simulink model "INtegrated_Simplified_Batteries_2"  (R2025a)
settings: Solver=ode113  StartTime=0.0  StopTime=20000  FixedStep=0.01  MaxStep=0.1  RelTol=1e-3
libraries: simulink x16, slpidlib x2, spsFirstOrderFilterLib x1
(part 2 of 3)

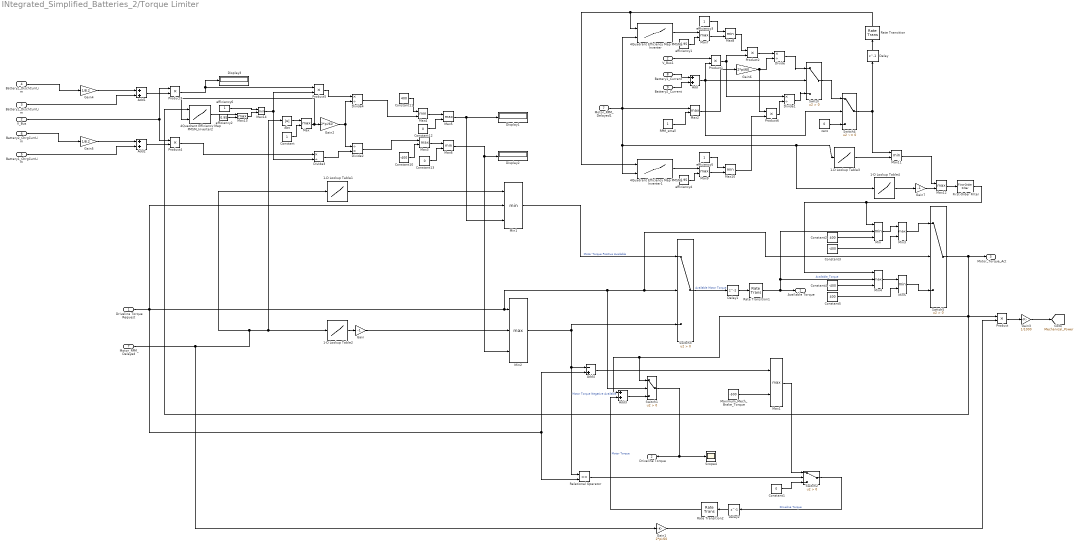
== system INtegrated_Simplified_Batteries_2/Torque Limiter ==
  Driveline Torque Request : Inport
  V_Bus : Inport  Port=2
  Battery1_DischCurrLim : Inport  Port=3
  Battery2_DischCurrLim : Inport  Port=4
  Battery1_ChrgCurrLim : Inport  Port=5
  Battery2_ChrgCurrLim : Inport  Port=6
  Motor_RPM_Delayed : Inport  Port=7
  Battery1_Current : Inport  Port=8
  Battery2_Current : Inport  Port=9
  1-D Lookup Table1 : Lookup_n-D  NumberOfTableDimensions=1  BreakpointsForDimension1=-19500:550:19500  Table=|  InternalRulePriority=Speed  RndMeth=Simplest
      | [5.617233286
      | 97.42737775
      | 101.4868518
      | 105.8188093
      | 110.4506091
      | 115.4133846
      | 120.7427184
      | 126.4794656
      | 132.6707681
      | 139.3713119
      | 146.6448989
      | 154.5664284
      | 163.2244193
      | 172.7242532
      | 183.1923898
      | 194.7819136
      | 207.6799304
      | 222.1175726
      | 238.3837585
      | 256.8444536
      | 277.9701878
      | 302.3762727
      | 330.8831267
      | 364.609506
      | 400
      | 400
      | 400
      | 400
      | 400
      | 400
      | 400
      | 400
      | 400
      | 400
      | 400
      | 400
      | 400
      | 400
      | 400
      | 400
      | 400
      | 400
      | 400
      | 400
      | 400
      | 400
      | 364.609506
      | 330.8831267
      | 302.3762727
      | 277.9701878
      | 256.8444536
      | 238.3837585
      | 222.1175726
      | 207.6799304
      | 194.7819136
      | 183.1923898
      | 172.7242532
      | 163.2244193
      | 154.5664284
      | 146.6448989
      | 139.3713119
      | 132.6707681
      | 126.4794656
      | 120.7427184
      | 115.4133846
      | 110.4506091
      | 105.8188093
      | 101.4868518
      | 97.42737775
      | 5.617233286
      | 0
      | ]
  1-D Lookup Table2 : Lookup_n-D  NumberOfTableDimensions=1  BreakpointsForDimension1=-19500:550:19500  Table=|  InternalRulePriority=Speed  RndMeth=Simplest
      | [5.617233286
      | 97.42737775
      | 101.4868518
      | 105.8188093
      | 110.4506091
      | 115.4133846
      | 120.7427184
      | 126.4794656
      | 132.6707681
      | 139.3713119
      | 146.6448989
      | 154.5664284
      | 163.2244193
      | 172.7242532
      | 183.1923898
      | 194.7819136
      | 207.6799304
      | 222.1175726
      | 238.3837585
      | 256.8444536
      | 277.9701878
      | 302.3762727
      | 330.8831267
      | 364.609506
      | 400
      | 400
      | 400
      | 400
      | 400
      | 400
      | 400
      | 400
      | 400
      | 400
      | 400
      | 400
      | 400
      | 400
      | 400
      | 400
      | 400
      | 400
      | 400
      | 400
      | 400
      | 400
      | 364.609506
      | 330.8831267
      | 302.3762727
      | 277.9701878
      | 256.8444536
      | 238.3837585
      | 222.1175726
      | 207.6799304
      | 194.7819136
      | 183.1923898
      | 172.7242532
      | 163.2244193
      | 154.5664284
      | 146.6448989
      | 139.3713119
      | 132.6707681
      | 126.4794656
      | 120.7427184
      | 115.4133846
      | 110.4506091
      | 105.8188093
      | 101.4868518
      | 97.42737775
      | 5.617233286
      | 0
      | ]
  1-D Lookup Table3 : Lookup_n-D  NumberOfTableDimensions=1  BreakpointsForDimension1=-19500:550:19500  Table=|  InternalRulePriority=Speed  RndMeth=Simplest
      | [5.617233286
      | 97.42737775
      | 101.4868518
      | 105.8188093
      | 110.4506091
      | 115.4133846
      | 120.7427184
      | 126.4794656
      | 132.6707681
      | 139.3713119
      | 146.6448989
      | 154.5664284
      | 163.2244193
      | 172.7242532
      | 183.1923898
      | 194.7819136
      | 207.6799304
      | 222.1175726
      | 238.3837585
      | 256.8444536
      | 277.9701878
      | 302.3762727
      | 330.8831267
      | 364.609506
      | 400
      | 400
      | 400
      | 400
      | 400
      | 400
      | 400
      | 400
      | 400
      | 400
      | 400
      | 400
      | 400
      | 400
      | 400
      | 400
      | 400
      | 400
      | 400
      | 400
      | 400
      | 400
      | 364.609506
      | 330.8831267
      | 302.3762727
      | 277.9701878
      | 256.8444536
      | 238.3837585
      | 222.1175726
      | 207.6799304
      | 194.7819136
      | 183.1923898
      | 172.7242532
      | 163.2244193
      | 154.5664284
      | 146.6448989
      | 139.3713119
      | 132.6707681
      | 126.4794656
      | 120.7427184
      | 115.4133846
      | 110.4506091
      | 105.8188093
      | 101.4868518
      | 97.42737775
      | 5.617233286
      | 0
      | ]
  1-D Lookup Table4 : Lookup_n-D  NumberOfTableDimensions=1  BreakpointsForDimension1=-19500:550:19500  Table=|  InternalRulePriority=Speed  RndMeth=Simplest
      | [5.617233286
      | 97.42737775
      | 101.4868518
      | 105.8188093
      | 110.4506091
      | 115.4133846
      | 120.7427184
      | 126.4794656
      | 132.6707681
      | 139.3713119
      | 146.6448989
      | 154.5664284
      | 163.2244193
      | 172.7242532
      | 183.1923898
      | 194.7819136
      | 207.6799304
      | 222.1175726
      | 238.3837585
      | 256.8444536
      | 277.9701878
      | 302.3762727
      | 330.8831267
      | 364.609506
      | 400
      | 400
      | 400
      | 400
      | 400
      | 400
      | 400
      | 400
      | 400
      | 400
      | 400
      | 400
      | 400
      | 400
      | 400
      | 400
      | 400
      | 400
      | 400
      | 400
      | 400
      | 400
      | 364.609506
      | 330.8831267
      | 302.3762727
      | 277.9701878
      | 256.8444536
      | 238.3837585
      | 222.1175726
      | 207.6799304
      | 194.7819136
      | 183.1923898
      | 172.7242532
      | 163.2244193
      | 154.5664284
      | 146.6448989
      | 139.3713119
      | 132.6707681
      | 126.4794656
      | 120.7427184
      | 115.4133846
      | 110.4506091
      | 105.8188093
      | 101.4868518
      | 97.42737775
      | 5.617233286
      | 0
      | ]
  4Quadrant Efficiency Map PMSM_Inverter : Lookup_n-D  BreakpointsForDimension1=-200:20:200  BreakpointsForDimension2=-16000:500:16000  Table=|  InterpMethod=Akima spline  InternalRulePriority=Speed  RndMeth=Simplest
      | [0.9785 0.9788 0.9792 0.9795 0.9799 0.9800 0.9800 0.9800 0.9800 0.9800 0.9800 0.9800 0.9800 0.9800 0.9800 0.9800 0.9800 0.9800 0.9800 0.9800 0.9800 0.9800 0.9800 0.9794 0.9781 0.9762 0.9737 0.9699 0.9641 0.9542 0.9347 0.8797 0.0000 0.8632 0.9301 0.9520 0.9628 0.9690 0.9730 0.9757 0.9776 0.9789 0.9799 0.9800 0.9800 0.9800 0.9800 0.9800 0.9800 0.9800 0.9800 0.9800 0.9800 0.9800 0.9800 0.9800 0.9800 0.9800 0.9800 0.9798 0.9794 0.9791 0.9787 0.9784 0.9780;
      | 0.9770 0.9774 0.9778 0.9782 0.9786 0.9790 0.9794 0.9797 0.9800 0.9800 0.9800 0.9800 0.9800 0.9800 0.9800 0.9800 0.9800 0.9800 0.9800 0.9800 0.9800 0.9800 0.9800 0.9800 0.9790 0.9774 0.9752 0.9719 0.9667 0.9578 0.9400 0.8894 0.0000 0.8756 0.9361 0.9559 0.9655 0.9711 0.9746 0.9769 0.9785 0.9797 0.9800 0.9800 0.9800 0.9800 0.9800 0.9800 0.9800 0.9800 0.9800 0.9800 0.9800 0.9800 0.9800 0.9797 0.9793 0.9789 0.9785 0.9781 0.9777 0.9773 0.9769 0.9764 0.9764;
      | 0.9750 0.9755 0.9760 0.9765 0.9769 0.9774 0.9779 0.9783 0.9787 0.9792 0.9796 0.9799 0.9800 0.9800 0.9800 0.9800 0.9800 0.9800 0.9800 0.9800 0.9800 0.9800 0.9800 0.9800 0.9797 0.9785 0.9766 0.9737 0.9691 0.9612 0.9452 0.8992 0.0000 0.8878 0.9420 0.9596 0.9681 0.9730 0.9760 0.9780 0.9793 0.9800 0.9800 0.9800 0.9800 0.9800 0.9800 0.9800 0.9800 0.9800 0.9800 0.9800 0.9799 0.9795 0.9791 0.9787 0.9783 0.9778 0.9774 0.9769 0.9764 0.9759 0.9754 0.9749 0.9743;
      | 0.9723 0.9729 0.9735 0.9741 0.9747 0.9752 0.9758 0.9764 0.9769 0.9774 0.9779 0.9784 0.9789 0.9793 0.9798 0.9800 0.9800 0.9800 0.9800 0.9800 0.9800 0.9800 0.9800 0.9800 0.9800 0.9793 0.9778 0.9754 0.9714 0.9645 0.9503 0.9089 0.0000 0.8998 0.9477 0.9632 0.9706 0.9747 0.9772 0.9788 0.9799 0.9800 0.9800 0.9800 0.9800 0.9800 0.9800 0.9800 0.9800 0.9798 0.9794 0.9789 0.9784 0.9779 0.9774 0.9769 0.9763 0.9758 0.9752 0.9746 0.9740 0.9734 0.9728 0.9722 0.9716;
      | 0.9687 0.9694 0.9701 0.9708 0.9715 0.9722 0.9729 0.9736 0.9743 0.9749 0.9756 0.9762 0.9768 0.9774 0.9780 0.9785 0.9790 0.9795 0.9799 0.9800 0.9800 0.9800 0.9800 0.9800 0.9800 0.9798 0.9786 0.9767 0.9735 0.9676 0.9553 0.9186 0.0000 0.9114 0.9532 0.9665 0.9728 0.9762 0.9782 0.9794 0.9800 0.9800 0.9800 0.9800 0.9800 0.9799 0.9795 0.9791 0.9786 0.9780 0.9775 0.9769 0.9763 0.9756 0.9750 0.9743 0.9736 0.9729 0.9722 0.9714 0.9707 0.9700 0.9692 0.9685 0.9677;
      | 0.9635 0.9644 0.9653 0.9661 0.9670 0.9679 0.9687 0.9696 0.9704 0.9712 0.9721 0.9729 0.9737 0.9744 0.9752 0.9759 0.9767 0.9773 0.9780 0.9786 0.9791 0.9795 0.9798 0.9800 0.9800 0.9798 0.9790 0.9777 0.9751 0.9703 0.9598 0.9280 0.0000 0.9224 0.9582 0.9694 0.9745 0.9772 0.9786 0.9793 0.9796 0.9796 0.9794 0.9791 0.9786 0.9781 0.9775 0.9768 0.9761 0.9753 0.9746 0.9738 0.9730 0.9721 0.9713 0.9704 0.9695 0.9686 0.9677 0.9668 0.9659 0.9649 0.9640 0.9631 0.9621;
      | 0.9557 0.9568 0.9579 0.9590 0.9601 0.9611 0.9622 0.9633 0.9644 0.9655 0.9666 0.9676 0.9687 0.9697 0.9707 0.9717 0.9727 0.9737 0.9746 0.9755 0.9763 0.9771 0.9777 0.9783 0.9787 0.9788 0.9786 0.9778 0.9761 0.9723 0.9638 0.9367 0.0000 0.9324 0.9624 0.9715 0.9755 0.9773 0.9781 0.9784 0.9782 0.9778 0.9772 0.9765 0.9757 0.9749 0.9739 0.9730 0.9720 0.9709 0.9699 0.9688 0.9677 0.9665 0.9654 0.9643 0.9631 0.9619 0.9608 0.9596 0.9584 0.9572 0.9560 0.9548 0.9536;
      | 0.9426 0.9440 0.9455 0.9470 0.9484 0.9499 0.9513 0.9528 0.9543 0.9557 0.9572 0.9586 0.9601 0.9615 0.9629 0.9643 0.9657 0.9671 0.9685 0.9698 0.9710 0.9723 0.9734 0.9745 0.9754 0.9761 0.9765 0.9764 0.9755 0.9730 0.9663 0.9438 0.0000 0.9404 0.9651 0.9722 0.9749 0.9759 0.9759 0.9755 0.9748 0.9738 0.9727 0.9715 0.9702 0.9688 0.9674 0.9660 0.9645 0.9630 0.9615 0.9600 0.9584 0.9568 0.9553 0.9537 0.9521 0.9505 0.9489 0.9472 0.9456 0.9440 0.9424 0.9407 0.9391;
      | 0.9171 0.9192 0.9213 0.9234 0.9256 0.9277 0.9298 0.9320 0.9341 0.9363 0.9384 0.9406 0.9427 0.9449 0.9470 0.9492 0.9513 0.9534 0.9555 0.9576 0.9597 0.9617 0.9637 0.9656 0.9673 0.9689 0.9703 0.9712 0.9714 0.9701 0.9653 0.9463 0.0000 0.9433 0.9640 0.9692 0.9706 0.9703 0.9694 0.9679 0.9662 0.9643 0.9623 0.9602 0.9580 0.9558 0.9535 0.9512 0.9488 0.9464 0.9441 0.9417 0.9392 0.9368 0.9344 0.9319 0.9295 0.9270 0.9245 0.9221 0.9196 0.9171 0.9146 0.9121 0.9096;
      | 0.8478 0.8514 0.8551 0.8588 0.8625 0.8662 0.8700 0.8738 0.8776 0.8815 0.8854 0.8893 0.8932 0.8972 0.9011 0.9051 0.9091 0.9132 0.9172 0.9213 0.9253 0.9293 0.9333 0.9372 0.9410 0.9447 0.9481 0.9510 0.9532 0.9537 0.9502 0.9309 0.0000 0.9257 0.9476 0.9515 0.9509 0.9485 0.9452 0.9415 0.9373 0.9330 0.9285 0.9239 0.9193 0.9145 0.9097 0.9049 0.9001 0.8952 0.8903 0.8854 0.8804 0.8755 0.8705 0.8655 0.8606 0.8556 0.8506 0.8456 0.8406 0.8356 0.8305 0.8255 0.8205;
      | 0.0000 0.0000 0.0000 0.0000 0.0000 0.0000 0.0000 0.0000 0.0000 0.0000 0.0000 0.0000 0.0000 0.0000 0.0000 0.0000 0.0000 0.0000 0.0000 0.0000 0.0000 0.0000 0.0000 0.0000 0.0000 0.0000 0.0000 0.0000 0.0000 0.0000 0.0000 0.0000 0.0000 0.0000 0.0000 0.0000 0.0000 0.0000 0.0000 0.0000 0.0000 0.0000 0.0000 0.0000 0.0000 0.0000 0.0000 0.0000 0.0000 0.0000 0.0000 0.0000 0.0000 0.0000 0.0000 0.0000 0.0000 0.0000 0.0000 0.0000 0.0000 0.0000 0.0000 0.0000 0.0000;
      | 0.8205 0.8255 0.8305 0.8356 0.8406 0.8456 0.8506 0.8556 0.8606 0.8655 0.8705 0.8755 0.8804 0.8854 0.8903 0.8952 0.9001 0.9049 0.9097 0.9145 0.9193 0.9239 0.9285 0.9330 0.9373 0.9415 0.9452 0.9485 0.9509 0.9515 0.9476 0.9257 0.0000 0.9309 0.9502 0.9537 0.9532 0.9510 0.9481 0.9447 0.9410 0.9372 0.9333 0.9293 0.9253 0.9213 0.9172 0.9132 0.9091 0.9051 0.9011 0.8972 0.8932 0.8893 0.8854 0.8815 0.8776 0.8738 0.8700 0.8662 0.8625 0.8588 0.8551 0.8514 0.8478;
      | 0.9096 0.9121 0.9146 0.9171 0.9196 0.9221 0.9245 0.9270 0.9295 0.9319 0.9344 0.9368 0.9392 0.9417 0.9441 0.9464 0.9488 0.9512 0.9535 0.9558 0.9580 0.9602 0.9623 0.9643 0.9662 0.9679 0.9694 0.9703 0.9706 0.9692 0.9640 0.9433 0.0000 0.9463 0.9653 0.9701 0.9714 0.9712 0.9703 0.9689 0.9673 0.9656 0.9637 0.9617 0.9597 0.9576 0.9555 0.9534 0.9513 0.9492 0.9470 0.9449 0.9427 0.9406 0.9384 0.9363 0.9341 0.9320 0.9298 0.9277 0.9256 0.9234 0.9213 0.9192 0.9171;
      | 0.9391 0.9407 0.9424 0.9440 0.9456 0.9472 0.9489 0.9505 0.9521 0.9537 0.9553 0.9568 0.9584 0.9600 0.9615 0.9630 0.9645 0.9660 0.9674 0.9688 0.9702 0.9715 0.9727 0.9738 0.9748 0.9755 0.9759 0.9759 0.9749 0.9722 0.9651 0.9404 0.0000 0.9438 0.9663 0.9730 0.9755 0.9764 0.9765 0.9761 0.9754 0.9745 0.9734 0.9723 0.9710 0.9698 0.9685 0.9671 0.9657 0.9643 0.9629 0.9615 0.9601 0.9586 0.9572 0.9557 0.9543 0.9528 0.9513 0.9499 0.9484 0.9470 0.9455 0.9440 0.9426;
      | 0.9536 0.9548 0.9560 0.9572 0.9584 0.9596 0.9608 0.9619 0.9631 0.9643 0.9654 0.9665 0.9677 0.9688 0.9699 0.9709 0.9720 0.9730 0.9739 0.9749 0.9757 0.9765 0.9772 0.9778 0.9782 0.9784 0.9781 0.9773 0.9755 0.9715 0.9624 0.9324 0.0000 0.9367 0.9638 0.9723 0.9761 0.9778 0.9786 0.9788 0.9787 0.9783 0.9777 0.9771 0.9763 0.9755 0.9746 0.9737 0.9727 0.9717 0.9707 0.9697 0.9687 0.9676 0.9666 0.9655 0.9644 0.9633 0.9622 0.9611 0.9601 0.9590 0.9579 0.9568 0.9557;
      | 0.9621 0.9631 0.9640 0.9649 0.9659 0.9668 0.9677 0.9686 0.9695 0.9704 0.9713 0.9721 0.9730 0.9738 0.9746 0.9753 0.9761 0.9768 0.9775 0.9781 0.9786 0.9791 0.9794 0.9796 0.9796 0.9793 0.9786 0.9772 0.9745 0.9694 0.9582 0.9224 0.0000 0.9280 0.9598 0.9703 0.9751 0.9777 0.9790 0.9798 0.9800 0.9800 0.9798 0.9795 0.9791 0.9786 0.9780 0.9773 0.9767 0.9759 0.9752 0.9744 0.9737 0.9729 0.9721 0.9712 0.9704 0.9696 0.9687 0.9679 0.9670 0.9661 0.9653 0.9644 0.9635;
      | 0.9677 0.9685 0.9692 0.9700 0.9707 0.9714 0.9722 0.9729 0.9736 0.9743 0.9750 0.9756 0.9763 0.9769 0.9775 0.9780 0.9786 0.9791 0.9795 0.9799 0.9800 0.9800 0.9800 0.9800 0.9800 0.9794 0.9782 0.9762 0.9728 0.9665 0.9532 0.9114 0.0000 0.9186 0.9553 0.9676 0.9735 0.9767 0.9786 0.9798 0.9800 0.9800 0.9800 0.9800 0.9800 0.9800 0.9799 0.9795 0.9790 0.9785 0.9780 0.9774 0.9768 0.9762 0.9756 0.9749 0.9743 0.9736 0.9729 0.9722 0.9715 0.9708 0.9701 0.9694 0.9687;
      | 0.9716 0.9722 0.9728 0.9734 0.9740 0.9746 0.9752 0.9758 0.9763 0.9769 0.9774 0.9779 0.9784 0.9789 0.9794 0.9798 0.9800 0.9800 0.9800 0.9800 0.9800 0.9800 0.9800 0.9800 0.9799 0.9788 0.9772 0.9747 0.9706 0.9632 0.9477 0.8998 0.0000 0.9089 0.9503 0.9645 0.9714 0.9754 0.9778 0.9793 0.9800 0.9800 0.9800 0.9800 0.9800 0.9800 0.9800 0.9800 0.9800 0.9800 0.9798 0.9793 0.9789 0.9784 0.9779 0.9774 0.9769 0.9764 0.9758 0.9752 0.9747 0.9741 0.9735 0.9729 0.9723;
      | 0.9743 0.9749 0.9754 0.9759 0.9764 0.9769 0.9774 0.9778 0.9783 0.9787 0.9791 0.9795 0.9799 0.9800 0.9800 0.9800 0.9800 0.9800 0.9800 0.9800 0.9800 0.9800 0.9800 0.9800 0.9793 0.9780 0.9760 0.9730 0.9681 0.9596 0.9420 0.8878 0.0000 0.8992 0.9452 0.9612 0.9691 0.9737 0.9766 0.9785 0.9797 0.9800 0.9800 0.9800 0.9800 0.9800 0.9800 0.9800 0.9800 0.9800 0.9800 0.9800 0.9800 0.9799 0.9796 0.9792 0.9787 0.9783 0.9779 0.9774 0.9769 0.9765 0.9760 0.9755 0.9750;
      | 0.9764 0.9769 0.9773 0.9777 0.9781 0.9785 0.9789 0.9793 0.9797 0.9800 0.9800 0.9800 0.9800 0.9800 0.9800 0.9800 0.9800 0.9800 0.9800 0.9800 0.9800 0.9800 0.9800 0.9797 0.9785 0.9769 0.9746 0.9711 0.9655 0.9559 0.9361 0.8756 0.0000 0.8894 0.9400 0.9578 0.9667 0.9719 0.9752 0.9774 0.9790 0.9800 0.9800 0.9800 0.9800 0.9800 0.9800 0.9800 0.9800 0.9800 0.9800 0.9800 0.9800 0.9800 0.9800 0.9800 0.9800 0.9797 0.9794 0.9790 0.9786 0.9782 0.9778 0.9774 0.9770;
      | 0.9780 0.9784 0.9787 0.9791 0.9794 0.9798 0.9800 0.9800 0.9800 0.9800 0.9800 0.9800 0.9800 0.9800 0.9800 0.9800 0.9800 0.9800 0.9800 0.9800 0.9800 0.9800 0.9799 0.9789 0.9776 0.9757 0.9730 0.9690 0.9628 0.9520 0.9301 0.8632 0.0000 0.8797 0.9347 0.9542 0.9641 0.9699 0.9737 0.9762 0.9781 0.9794 0.9800 0.9800 0.9800 0.9800 0.9800 0.9800 0.9800 0.9800 0.9800 0.9800 0.9800 0.9800 0.9800 0.9800 0.9800 0.9800 0.9800 0.9800 0.9799 0.9795 0.9792 0.9788 0.9785];
      settings: InputPortMap=u0,u1
  4Quadrant Efficiency Map PMSM_Inverter1 : Lookup_n-D  BreakpointsForDimension1=-200:20:200  BreakpointsForDimension2=-16000:500:16000  Table=|  InterpMethod=Akima spline  InternalRulePriority=Speed  RndMeth=Simplest
      | [0.9785 0.9788 0.9792 0.9795 0.9799 0.9800 0.9800 0.9800 0.9800 0.9800 0.9800 0.9800 0.9800 0.9800 0.9800 0.9800 0.9800 0.9800 0.9800 0.9800 0.9800 0.9800 0.9800 0.9794 0.9781 0.9762 0.9737 0.9699 0.9641 0.9542 0.9347 0.8797 0.0000 0.8632 0.9301 0.9520 0.9628 0.9690 0.9730 0.9757 0.9776 0.9789 0.9799 0.9800 0.9800 0.9800 0.9800 0.9800 0.9800 0.9800 0.9800 0.9800 0.9800 0.9800 0.9800 0.9800 0.9800 0.9800 0.9800 0.9798 0.9794 0.9791 0.9787 0.9784 0.9780;
      | 0.9770 0.9774 0.9778 0.9782 0.9786 0.9790 0.9794 0.9797 0.9800 0.9800 0.9800 0.9800 0.9800 0.9800 0.9800 0.9800 0.9800 0.9800 0.9800 0.9800 0.9800 0.9800 0.9800 0.9800 0.9790 0.9774 0.9752 0.9719 0.9667 0.9578 0.9400 0.8894 0.0000 0.8756 0.9361 0.9559 0.9655 0.9711 0.9746 0.9769 0.9785 0.9797 0.9800 0.9800 0.9800 0.9800 0.9800 0.9800 0.9800 0.9800 0.9800 0.9800 0.9800 0.9800 0.9800 0.9797 0.9793 0.9789 0.9785 0.9781 0.9777 0.9773 0.9769 0.9764 0.9764;
      | 0.9750 0.9755 0.9760 0.9765 0.9769 0.9774 0.9779 0.9783 0.9787 0.9792 0.9796 0.9799 0.9800 0.9800 0.9800 0.9800 0.9800 0.9800 0.9800 0.9800 0.9800 0.9800 0.9800 0.9800 0.9797 0.9785 0.9766 0.9737 0.9691 0.9612 0.9452 0.8992 0.0000 0.8878 0.9420 0.9596 0.9681 0.9730 0.9760 0.9780 0.9793 0.9800 0.9800 0.9800 0.9800 0.9800 0.9800 0.9800 0.9800 0.9800 0.9800 0.9800 0.9799 0.9795 0.9791 0.9787 0.9783 0.9778 0.9774 0.9769 0.9764 0.9759 0.9754 0.9749 0.9743;
      | 0.9723 0.9729 0.9735 0.9741 0.9747 0.9752 0.9758 0.9764 0.9769 0.9774 0.9779 0.9784 0.9789 0.9793 0.9798 0.9800 0.9800 0.9800 0.9800 0.9800 0.9800 0.9800 0.9800 0.9800 0.9800 0.9793 0.9778 0.9754 0.9714 0.9645 0.9503 0.9089 0.0000 0.8998 0.9477 0.9632 0.9706 0.9747 0.9772 0.9788 0.9799 0.9800 0.9800 0.9800 0.9800 0.9800 0.9800 0.9800 0.9800 0.9798 0.9794 0.9789 0.9784 0.9779 0.9774 0.9769 0.9763 0.9758 0.9752 0.9746 0.9740 0.9734 0.9728 0.9722 0.9716;
      | 0.9687 0.9694 0.9701 0.9708 0.9715 0.9722 0.9729 0.9736 0.9743 0.9749 0.9756 0.9762 0.9768 0.9774 0.9780 0.9785 0.9790 0.9795 0.9799 0.9800 0.9800 0.9800 0.9800 0.9800 0.9800 0.9798 0.9786 0.9767 0.9735 0.9676 0.9553 0.9186 0.0000 0.9114 0.9532 0.9665 0.9728 0.9762 0.9782 0.9794 0.9800 0.9800 0.9800 0.9800 0.9800 0.9799 0.9795 0.9791 0.9786 0.9780 0.9775 0.9769 0.9763 0.9756 0.9750 0.9743 0.9736 0.9729 0.9722 0.9714 0.9707 0.9700 0.9692 0.9685 0.9677;
      | 0.9635 0.9644 0.9653 0.9661 0.9670 0.9679 0.9687 0.9696 0.9704 0.9712 0.9721 0.9729 0.9737 0.9744 0.9752 0.9759 0.9767 0.9773 0.9780 0.9786 0.9791 0.9795 0.9798 0.9800 0.9800 0.9798 0.9790 0.9777 0.9751 0.9703 0.9598 0.9280 0.0000 0.9224 0.9582 0.9694 0.9745 0.9772 0.9786 0.9793 0.9796 0.9796 0.9794 0.9791 0.9786 0.9781 0.9775 0.9768 0.9761 0.9753 0.9746 0.9738 0.9730 0.9721 0.9713 0.9704 0.9695 0.9686 0.9677 0.9668 0.9659 0.9649 0.9640 0.9631 0.9621;
      | 0.9557 0.9568 0.9579 0.9590 0.9601 0.9611 0.9622 0.9633 0.9644 0.9655 0.9666 0.9676 0.9687 0.9697 0.9707 0.9717 0.9727 0.9737 0.9746 0.9755 0.9763 0.9771 0.9777 0.9783 0.9787 0.9788 0.9786 0.9778 0.9761 0.9723 0.9638 0.9367 0.0000 0.9324 0.9624 0.9715 0.9755 0.9773 0.9781 0.9784 0.9782 0.9778 0.9772 0.9765 0.9757 0.9749 0.9739 0.9730 0.9720 0.9709 0.9699 0.9688 0.9677 0.9665 0.9654 0.9643 0.9631 0.9619 0.9608 0.9596 0.9584 0.9572 0.9560 0.9548 0.9536;
      | 0.9426 0.9440 0.9455 0.9470 0.9484 0.9499 0.9513 0.9528 0.9543 0.9557 0.9572 0.9586 0.9601 0.9615 0.9629 0.9643 0.9657 0.9671 0.9685 0.9698 0.9710 0.9723 0.9734 0.9745 0.9754 0.9761 0.9765 0.9764 0.9755 0.9730 0.9663 0.9438 0.0000 0.9404 0.9651 0.9722 0.9749 0.9759 0.9759 0.9755 0.9748 0.9738 0.9727 0.9715 0.9702 0.9688 0.9674 0.9660 0.9645 0.9630 0.9615 0.9600 0.9584 0.9568 0.9553 0.9537 0.9521 0.9505 0.9489 0.9472 0.9456 0.9440 0.9424 0.9407 0.9391;
      | 0.9171 0.9192 0.9213 0.9234 0.9256 0.9277 0.9298 0.9320 0.9341 0.9363 0.9384 0.9406 0.9427 0.9449 0.9470 0.9492 0.9513 0.9534 0.9555 0.9576 0.9597 0.9617 0.9637 0.9656 0.9673 0.9689 0.9703 0.9712 0.9714 0.9701 0.9653 0.9463 0.0000 0.9433 0.9640 0.9692 0.9706 0.9703 0.9694 0.9679 0.9662 0.9643 0.9623 0.9602 0.9580 0.9558 0.9535 0.9512 0.9488 0.9464 0.9441 0.9417 0.9392 0.9368 0.9344 0.9319 0.9295 0.9270 0.9245 0.9221 0.9196 0.9171 0.9146 0.9121 0.9096;
      | 0.8478 0.8514 0.8551 0.8588 0.8625 0.8662 0.8700 0.8738 0.8776 0.8815 0.8854 0.8893 0.8932 0.8972 0.9011 0.9051 0.9091 0.9132 0.9172 0.9213 0.9253 0.9293 0.9333 0.9372 0.9410 0.9447 0.9481 0.9510 0.9532 0.9537 0.9502 0.9309 0.0000 0.9257 0.9476 0.9515 0.9509 0.9485 0.9452 0.9415 0.9373 0.9330 0.9285 0.9239 0.9193 0.9145 0.9097 0.9049 0.9001 0.8952 0.8903 0.8854 0.8804 0.8755 0.8705 0.8655 0.8606 0.8556 0.8506 0.8456 0.8406 0.8356 0.8305 0.8255 0.8205;
      | 0.0000 0.0000 0.0000 0.0000 0.0000 0.0000 0.0000 0.0000 0.0000 0.0000 0.0000 0.0000 0.0000 0.0000 0.0000 0.0000 0.0000 0.0000 0.0000 0.0000 0.0000 0.0000 0.0000 0.0000 0.0000 0.0000 0.0000 0.0000 0.0000 0.0000 0.0000 0.0000 0.0000 0.0000 0.0000 0.0000 0.0000 0.0000 0.0000 0.0000 0.0000 0.0000 0.0000 0.0000 0.0000 0.0000 0.0000 0.0000 0.0000 0.0000 0.0000 0.0000 0.0000 0.0000 0.0000 0.0000 0.0000 0.0000 0.0000 0.0000 0.0000 0.0000 0.0000 0.0000 0.0000;
      | 0.8205 0.8255 0.8305 0.8356 0.8406 0.8456 0.8506 0.8556 0.8606 0.8655 0.8705 0.8755 0.8804 0.8854 0.8903 0.8952 0.9001 0.9049 0.9097 0.9145 0.9193 0.9239 0.9285 0.9330 0.9373 0.9415 0.9452 0.9485 0.9509 0.9515 0.9476 0.9257 0.0000 0.9309 0.9502 0.9537 0.9532 0.9510 0.9481 0.9447 0.9410 0.9372 0.9333 0.9293 0.9253 0.9213 0.9172 0.9132 0.9091 0.9051 0.9011 0.8972 0.8932 0.8893 0.8854 0.8815 0.8776 0.8738 0.8700 0.8662 0.8625 0.8588 0.8551 0.8514 0.8478;
      | 0.9096 0.9121 0.9146 0.9171 0.9196 0.9221 0.9245 0.9270 0.9295 0.9319 0.9344 0.9368 0.9392 0.9417 0.9441 0.9464 0.9488 0.9512 0.9535 0.9558 0.9580 0.9602 0.9623 0.9643 0.9662 0.9679 0.9694 0.9703 0.9706 0.9692 0.9640 0.9433 0.0000 0.9463 0.9653 0.9701 0.9714 0.9712 0.9703 0.9689 0.9673 0.9656 0.9637 0.9617 0.9597 0.9576 0.9555 0.9534 0.9513 0.9492 0.9470 0.9449 0.9427 0.9406 0.9384 0.9363 0.9341 0.9320 0.9298 0.9277 0.9256 0.9234 0.9213 0.9192 0.9171;
      | 0.9391 0.9407 0.9424 0.9440 0.9456 0.9472 0.9489 0.9505 0.9521 0.9537 0.9553 0.9568 0.9584 0.9600 0.9615 0.9630 0.9645 0.9660 0.9674 0.9688 0.9702 0.9715 0.9727 0.9738 0.9748 0.9755 0.9759 0.9759 0.9749 0.9722 0.9651 0.9404 0.0000 0.9438 0.9663 0.9730 0.9755 0.9764 0.9765 0.9761 0.9754 0.9745 0.9734 0.9723 0.9710 0.9698 0.9685 0.9671 0.9657 0.9643 0.9629 0.9615 0.9601 0.9586 0.9572 0.9557 0.9543 0.9528 0.9513 0.9499 0.9484 0.9470 0.9455 0.9440 0.9426;
      | 0.9536 0.9548 0.9560 0.9572 0.9584 0.9596 0.9608 0.9619 0.9631 0.9643 0.9654 0.9665 0.9677 0.9688 0.9699 0.9709 0.9720 0.9730 0.9739 0.9749 0.9757 0.9765 0.9772 0.9778 0.9782 0.9784 0.9781 0.9773 0.9755 0.9715 0.9624 0.9324 0.0000 0.9367 0.9638 0.9723 0.9761 0.9778 0.9786 0.9788 0.9787 0.9783 0.9777 0.9771 0.9763 0.9755 0.9746 0.9737 0.9727 0.9717 0.9707 0.9697 0.9687 0.9676 0.9666 0.9655 0.9644 0.9633 0.9622 0.9611 0.9601 0.9590 0.9579 0.9568 0.9557;
      | 0.9621 0.9631 0.9640 0.9649 0.9659 0.9668 0.9677 0.9686 0.9695 0.9704 0.9713 0.9721 0.9730 0.9738 0.9746 0.9753 0.9761 0.9768 0.9775 0.9781 0.9786 0.9791 0.9794 0.9796 0.9796 0.9793 0.9786 0.9772 0.9745 0.9694 0.9582 0.9224 0.0000 0.9280 0.9598 0.9703 0.9751 0.9777 0.9790 0.9798 0.9800 0.9800 0.9798 0.9795 0.9791 0.9786 0.9780 0.9773 0.9767 0.9759 0.9752 0.9744 0.9737 0.9729 0.9721 0.9712 0.9704 0.9696 0.9687 0.9679 0.9670 0.9661 0.9653 0.9644 0.9635;
      | 0.9677 0.9685 0.9692 0.9700 0.9707 0.9714 0.9722 0.9729 0.9736 0.9743 0.9750 0.9756 0.9763 0.9769 0.9775 0.9780 0.9786 0.9791 0.9795 0.9799 0.9800 0.9800 0.9800 0.9800 0.9800 0.9794 0.9782 0.9762 0.9728 0.9665 0.9532 0.9114 0.0000 0.9186 0.9553 0.9676 0.9735 0.9767 0.9786 0.9798 0.9800 0.9800 0.9800 0.9800 0.9800 0.9800 0.9799 0.9795 0.9790 0.9785 0.9780 0.9774 0.9768 0.9762 0.9756 0.9749 0.9743 0.9736 0.9729 0.9722 0.9715 0.9708 0.9701 0.9694 0.9687;
      | 0.9716 0.9722 0.9728 0.9734 0.9740 0.9746 0.9752 0.9758 0.9763 0.9769 0.9774 0.9779 0.9784 0.9789 0.9794 0.9798 0.9800 0.9800 0.9800 0.9800 0.9800 0.9800 0.9800 0.9800 0.9799 0.9788 0.9772 0.9747 0.9706 0.9632 0.9477 0.8998 0.0000 0.9089 0.9503 0.9645 0.9714 0.9754 0.9778 0.9793 0.9800 0.9800 0.9800 0.9800 0.9800 0.9800 0.9800 0.9800 0.9800 0.9800 0.9798 0.9793 0.9789 0.9784 0.9779 0.9774 0.9769 0.9764 0.9758 0.9752 0.9747 0.9741 0.9735 0.9729 0.9723;
      | 0.9743 0.9749 0.9754 0.9759 0.9764 0.9769 0.9774 0.9778 0.9783 0.9787 0.9791 0.9795 0.9799 0.9800 0.9800 0.9800 0.9800 0.9800 0.9800 0.9800 0.9800 0.9800 0.9800 0.9800 0.9793 0.9780 0.9760 0.9730 0.9681 0.9596 0.9420 0.8878 0.0000 0.8992 0.9452 0.9612 0.9691 0.9737 0.9766 0.9785 0.9797 0.9800 0.9800 0.9800 0.9800 0.9800 0.9800 0.9800 0.9800 0.9800 0.9800 0.9800 0.9800 0.9799 0.9796 0.9792 0.9787 0.9783 0.9779 0.9774 0.9769 0.9765 0.9760 0.9755 0.9750;
      | 0.9764 0.9769 0.9773 0.9777 0.9781 0.9785 0.9789 0.9793 0.9797 0.9800 0.9800 0.9800 0.9800 0.9800 0.9800 0.9800 0.9800 0.9800 0.9800 0.9800 0.9800 0.9800 0.9800 0.9797 0.9785 0.9769 0.9746 0.9711 0.9655 0.9559 0.9361 0.8756 0.0000 0.8894 0.9400 0.9578 0.9667 0.9719 0.9752 0.9774 0.9790 0.9800 0.9800 0.9800 0.9800 0.9800 0.9800 0.9800 0.9800 0.9800 0.9800 0.9800 0.9800 0.9800 0.9800 0.9800 0.9800 0.9797 0.9794 0.9790 0.9786 0.9782 0.9778 0.9774 0.9770;
      | 0.9780 0.9784 0.9787 0.9791 0.9794 0.9798 0.9800 0.9800 0.9800 0.9800 0.9800 0.9800 0.9800 0.9800 0.9800 0.9800 0.9800 0.9800 0.9800 0.9800 0.9800 0.9800 0.9799 0.9789 0.9776 0.9757 0.9730 0.9690 0.9628 0.9520 0.9301 0.8632 0.0000 0.8797 0.9347 0.9542 0.9641 0.9699 0.9737 0.9762 0.9781 0.9794 0.9800 0.9800 0.9800 0.9800 0.9800 0.9800 0.9800 0.9800 0.9800 0.9800 0.9800 0.9800 0.9800 0.9800 0.9800 0.9800 0.9800 0.9800 0.9799 0.9795 0.9792 0.9788 0.9785];
      settings: InputPortMap=u0,u1
  4Quadrant Efficiency Map PMSM_Inverter2 : Lookup_n-D  BreakpointsForDimension1=-200:20:200  BreakpointsForDimension2=-16000:500:16000  Table=|  InterpMethod=Akima spline  InternalRulePriority=Speed  RndMeth=Simplest
      | [0.9785 0.9788 0.9792 0.9795 0.9799 0.9800 0.9800 0.9800 0.9800 0.9800 0.9800 0.9800 0.9800 0.9800 0.9800 0.9800 0.9800 0.9800 0.9800 0.9800 0.9800 0.9800 0.9800 0.9794 0.9781 0.9762 0.9737 0.9699 0.9641 0.9542 0.9347 0.8797 0.0000 0.8632 0.9301 0.9520 0.9628 0.9690 0.9730 0.9757 0.9776 0.9789 0.9799 0.9800 0.9800 0.9800 0.9800 0.9800 0.9800 0.9800 0.9800 0.9800 0.9800 0.9800 0.9800 0.9800 0.9800 0.9800 0.9800 0.9798 0.9794 0.9791 0.9787 0.9784 0.9780;
      | 0.9770 0.9774 0.9778 0.9782 0.9786 0.9790 0.9794 0.9797 0.9800 0.9800 0.9800 0.9800 0.9800 0.9800 0.9800 0.9800 0.9800 0.9800 0.9800 0.9800 0.9800 0.9800 0.9800 0.9800 0.9790 0.9774 0.9752 0.9719 0.9667 0.9578 0.9400 0.8894 0.0000 0.8756 0.9361 0.9559 0.9655 0.9711 0.9746 0.9769 0.9785 0.9797 0.9800 0.9800 0.9800 0.9800 0.9800 0.9800 0.9800 0.9800 0.9800 0.9800 0.9800 0.9800 0.9800 0.9797 0.9793 0.9789 0.9785 0.9781 0.9777 0.9773 0.9769 0.9764 0.9764;
      | 0.9750 0.9755 0.9760 0.9765 0.9769 0.9774 0.9779 0.9783 0.9787 0.9792 0.9796 0.9799 0.9800 0.9800 0.9800 0.9800 0.9800 0.9800 0.9800 0.9800 0.9800 0.9800 0.9800 0.9800 0.9797 0.9785 0.9766 0.9737 0.9691 0.9612 0.9452 0.8992 0.0000 0.8878 0.9420 0.9596 0.9681 0.9730 0.9760 0.9780 0.9793 0.9800 0.9800 0.9800 0.9800 0.9800 0.9800 0.9800 0.9800 0.9800 0.9800 0.9800 0.9799 0.9795 0.9791 0.9787 0.9783 0.9778 0.9774 0.9769 0.9764 0.9759 0.9754 0.9749 0.9743;
      | 0.9723 0.9729 0.9735 0.9741 0.9747 0.9752 0.9758 0.9764 0.9769 0.9774 0.9779 0.9784 0.9789 0.9793 0.9798 0.9800 0.9800 0.9800 0.9800 0.9800 0.9800 0.9800 0.9800 0.9800 0.9800 0.9793 0.9778 0.9754 0.9714 0.9645 0.9503 0.9089 0.0000 0.8998 0.9477 0.9632 0.9706 0.9747 0.9772 0.9788 0.9799 0.9800 0.9800 0.9800 0.9800 0.9800 0.9800 0.9800 0.9800 0.9798 0.9794 0.9789 0.9784 0.9779 0.9774 0.9769 0.9763 0.9758 0.9752 0.9746 0.9740 0.9734 0.9728 0.9722 0.9716;
      | 0.9687 0.9694 0.9701 0.9708 0.9715 0.9722 0.9729 0.9736 0.9743 0.9749 0.9756 0.9762 0.9768 0.9774 0.9780 0.9785 0.9790 0.9795 0.9799 0.9800 0.9800 0.9800 0.9800 0.9800 0.9800 0.9798 0.9786 0.9767 0.9735 0.9676 0.9553 0.9186 0.0000 0.9114 0.9532 0.9665 0.9728 0.9762 0.9782 0.9794 0.9800 0.9800 0.9800 0.9800 0.9800 0.9799 0.9795 0.9791 0.9786 0.9780 0.9775 0.9769 0.9763 0.9756 0.9750 0.9743 0.9736 0.9729 0.9722 0.9714 0.9707 0.9700 0.9692 0.9685 0.9677;
      | 0.9635 0.9644 0.9653 0.9661 0.9670 0.9679 0.9687 0.9696 0.9704 0.9712 0.9721 0.9729 0.9737 0.9744 0.9752 0.9759 0.9767 0.9773 0.9780 0.9786 0.9791 0.9795 0.9798 0.9800 0.9800 0.9798 0.9790 0.9777 0.9751 0.9703 0.9598 0.9280 0.0000 0.9224 0.9582 0.9694 0.9745 0.9772 0.9786 0.9793 0.9796 0.9796 0.9794 0.9791 0.9786 0.9781 0.9775 0.9768 0.9761 0.9753 0.9746 0.9738 0.9730 0.9721 0.9713 0.9704 0.9695 0.9686 0.9677 0.9668 0.9659 0.9649 0.9640 0.9631 0.9621;
      | 0.9557 0.9568 0.9579 0.9590 0.9601 0.9611 0.9622 0.9633 0.9644 0.9655 0.9666 0.9676 0.9687 0.9697 0.9707 0.9717 0.9727 0.9737 0.9746 0.9755 0.9763 0.9771 0.9777 0.9783 0.9787 0.9788 0.9786 0.9778 0.9761 0.9723 0.9638 0.9367 0.0000 0.9324 0.9624 0.9715 0.9755 0.9773 0.9781 0.9784 0.9782 0.9778 0.9772 0.9765 0.9757 0.9749 0.9739 0.9730 0.9720 0.9709 0.9699 0.9688 0.9677 0.9665 0.9654 0.9643 0.9631 0.9619 0.9608 0.9596 0.9584 0.9572 0.9560 0.9548 0.9536;
      | 0.9426 0.9440 0.9455 0.9470 0.9484 0.9499 0.9513 0.9528 0.9543 0.9557 0.9572 0.9586 0.9601 0.9615 0.9629 0.9643 0.9657 0.9671 0.9685 0.9698 0.9710 0.9723 0.9734 0.9745 0.9754 0.9761 0.9765 0.9764 0.9755 0.9730 0.9663 0.9438 0.0000 0.9404 0.9651 0.9722 0.9749 0.9759 0.9759 0.9755 0.9748 0.9738 0.9727 0.9715 0.9702 0.9688 0.9674 0.9660 0.9645 0.9630 0.9615 0.9600 0.9584 0.9568 0.9553 0.9537 0.9521 0.9505 0.9489 0.9472 0.9456 0.9440 0.9424 0.9407 0.9391;
      | 0.9171 0.9192 0.9213 0.9234 0.9256 0.9277 0.9298 0.9320 0.9341 0.9363 0.9384 0.9406 0.9427 0.9449 0.9470 0.9492 0.9513 0.9534 0.9555 0.9576 0.9597 0.9617 0.9637 0.9656 0.9673 0.9689 0.9703 0.9712 0.9714 0.9701 0.9653 0.9463 0.0000 0.9433 0.9640 0.9692 0.9706 0.9703 0.9694 0.9679 0.9662 0.9643 0.9623 0.9602 0.9580 0.9558 0.9535 0.9512 0.9488 0.9464 0.9441 0.9417 0.9392 0.9368 0.9344 0.9319 0.9295 0.9270 0.9245 0.9221 0.9196 0.9171 0.9146 0.9121 0.9096;
      | 0.8478 0.8514 0.8551 0.8588 0.8625 0.8662 0.8700 0.8738 0.8776 0.8815 0.8854 0.8893 0.8932 0.8972 0.9011 0.9051 0.9091 0.9132 0.9172 0.9213 0.9253 0.9293 0.9333 0.9372 0.9410 0.9447 0.9481 0.9510 0.9532 0.9537 0.9502 0.9309 0.0000 0.9257 0.9476 0.9515 0.9509 0.9485 0.9452 0.9415 0.9373 0.9330 0.9285 0.9239 0.9193 0.9145 0.9097 0.9049 0.9001 0.8952 0.8903 0.8854 0.8804 0.8755 0.8705 0.8655 0.8606 0.8556 0.8506 0.8456 0.8406 0.8356 0.8305 0.8255 0.8205;
      | 0.0000 0.0000 0.0000 0.0000 0.0000 0.0000 0.0000 0.0000 0.0000 0.0000 0.0000 0.0000 0.0000 0.0000 0.0000 0.0000 0.0000 0.0000 0.0000 0.0000 0.0000 0.0000 0.0000 0.0000 0.0000 0.0000 0.0000 0.0000 0.0000 0.0000 0.0000 0.0000 0.0000 0.0000 0.0000 0.0000 0.0000 0.0000 0.0000 0.0000 0.0000 0.0000 0.0000 0.0000 0.0000 0.0000 0.0000 0.0000 0.0000 0.0000 0.0000 0.0000 0.0000 0.0000 0.0000 0.0000 0.0000 0.0000 0.0000 0.0000 0.0000 0.0000 0.0000 0.0000 0.0000;
      | 0.8205 0.8255 0.8305 0.8356 0.8406 0.8456 0.8506 0.8556 0.8606 0.8655 0.8705 0.8755 0.8804 0.8854 0.8903 0.8952 0.9001 0.9049 0.9097 0.9145 0.9193 0.9239 0.9285 0.9330 0.9373 0.9415 0.9452 0.9485 0.9509 0.9515 0.9476 0.9257 0.0000 0.9309 0.9502 0.9537 0.9532 0.9510 0.9481 0.9447 0.9410 0.9372 0.9333 0.9293 0.9253 0.9213 0.9172 0.9132 0.9091 0.9051 0.9011 0.8972 0.8932 0.8893 0.8854 0.8815 0.8776 0.8738 0.8700 0.8662 0.8625 0.8588 0.8551 0.8514 0.8478;
      | 0.9096 0.9121 0.9146 0.9171 0.9196 0.9221 0.9245 0.9270 0.9295 0.9319 0.9344 0.9368 0.9392 0.9417 0.9441 0.9464 0.9488 0.9512 0.9535 0.9558 0.9580 0.9602 0.9623 0.9643 0.9662 0.9679 0.9694 0.9703 0.9706 0.9692 0.9640 0.9433 0.0000 0.9463 0.9653 0.9701 0.9714 0.9712 0.9703 0.9689 0.9673 0.9656 0.9637 0.9617 0.9597 0.9576 0.9555 0.9534 0.9513 0.9492 0.9470 0.9449 0.9427 0.9406 0.9384 0.9363 0.9341 0.9320 0.9298 0.9277 0.9256 0.9234 0.9213 0.9192 0.9171;
      | 0.9391 0.9407 0.9424 0.9440 0.9456 0.9472 0.9489 0.9505 0.9521 0.9537 0.9553 0.9568 0.9584 0.9600 0.9615 0.9630 0.9645 0.9660 0.9674 0.9688 0.9702 0.9715 0.9727 0.9738 0.9748 0.9755 0.9759 0.9759 0.9749 0.9722 0.9651 0.9404 0.0000 0.9438 0.9663 0.9730 0.9755 0.9764 0.9765 0.9761 0.9754 0.9745 0.9734 0.9723 0.9710 0.9698 0.9685 0.9671 0.9657 0.9643 0.9629 0.9615 0.9601 0.9586 0.9572 0.9557 0.9543 0.9528 0.9513 0.9499 0.9484 0.9470 0.9455 0.9440 0.9426;
      | 0.9536 0.9548 0.9560 0.9572 0.9584 0.9596 0.9608 0.9619 0.9631 0.9643 0.9654 0.9665 0.9677 0.9688 0.9699 0.9709 0.9720 0.9730 0.9739 0.9749 0.9757 0.9765 0.9772 0.9778 0.9782 0.9784 0.9781 0.9773 0.9755 0.9715 0.9624 0.9324 0.0000 0.9367 0.9638 0.9723 0.9761 0.9778 0.9786 0.9788 0.9787 0.9783 0.9777 0.9771 0.9763 0.9755 0.9746 0.9737 0.9727 0.9717 0.9707 0.9697 0.9687 0.9676 0.9666 0.9655 0.9644 0.9633 0.9622 0.9611 0.9601 0.9590 0.9579 0.9568 0.9557;
      | 0.9621 0.9631 0.9640 0.9649 0.9659 0.9668 0.9677 0.9686 0.9695 0.9704 0.9713 0.9721 0.9730 0.9738 0.9746 0.9753 0.9761 0.9768 0.9775 0.9781 0.9786 0.9791 0.9794 0.9796 0.9796 0.9793 0.9786 0.9772 0.9745 0.9694 0.9582 0.9224 0.0000 0.9280 0.9598 0.9703 0.9751 0.9777 0.9790 0.9798 0.9800 0.9800 0.9798 0.9795 0.9791 0.9786 0.9780 0.9773 0.9767 0.9759 0.9752 0.9744 0.9737 0.9729 0.9721 0.9712 0.9704 0.9696 0.9687 0.9679 0.9670 0.9661 0.9653 0.9644 0.9635;
      | 0.9677 0.9685 0.9692 0.9700 0.9707 0.9714 0.9722 0.9729 0.9736 0.9743 0.9750 0.9756 0.9763 0.9769 0.9775 0.9780 0.9786 0.9791 0.9795 0.9799 0.9800 0.9800 0.9800 0.9800 0.9800 0.9794 0.9782 0.9762 0.9728 0.9665 0.9532 0.9114 0.0000 0.9186 0.9553 0.9676 0.9735 0.9767 0.9786 0.9798 0.9800 0.9800 0.9800 0.9800 0.9800 0.9800 0.9799 0.9795 0.9790 0.9785 0.9780 0.9774 0.9768 0.9762 0.9756 0.9749 0.9743 0.9736 0.9729 0.9722 0.9715 0.9708 0.9701 0.9694 0.9687;
      | 0.9716 0.9722 0.9728 0.9734 0.9740 0.9746 0.9752 0.9758 0.9763 0.9769 0.9774 0.9779 0.9784 0.9789 0.9794 0.9798 0.9800 0.9800 0.9800 0.9800 0.9800 0.9800 0.9800 0.9800 0.9799 0.9788 0.9772 0.9747 0.9706 0.9632 0.9477 0.8998 0.0000 0.9089 0.9503 0.9645 0.9714 0.9754 0.9778 0.9793 0.9800 0.9800 0.9800 0.9800 0.9800 0.9800 0.9800 0.9800 0.9800 0.9800 0.9798 0.9793 0.9789 0.9784 0.9779 0.9774 0.9769 0.9764 0.9758 0.9752 0.9747 0.9741 0.9735 0.9729 0.9723;
      | 0.9743 0.9749 0.9754 0.9759 0.9764 0.9769 0.9774 0.9778 0.9783 0.9787 0.9791 0.9795 0.9799 0.9800 0.9800 0.9800 0.9800 0.9800 0.9800 0.9800 0.9800 0.9800 0.9800 0.9800 0.9793 0.9780 0.9760 0.9730 0.9681 0.9596 0.9420 0.8878 0.0000 0.8992 0.9452 0.9612 0.9691 0.9737 0.9766 0.9785 0.9797 0.9800 0.9800 0.9800 0.9800 0.9800 0.9800 0.9800 0.9800 0.9800 0.9800 0.9800 0.9800 0.9799 0.9796 0.9792 0.9787 0.9783 0.9779 0.9774 0.9769 0.9765 0.9760 0.9755 0.9750;
      | 0.9764 0.9769 0.9773 0.9777 0.9781 0.9785 0.9789 0.9793 0.9797 0.9800 0.9800 0.9800 0.9800 0.9800 0.9800 0.9800 0.9800 0.9800 0.9800 0.9800 0.9800 0.9800 0.9800 0.9797 0.9785 0.9769 0.9746 0.9711 0.9655 0.9559 0.9361 0.8756 0.0000 0.8894 0.9400 0.9578 0.9667 0.9719 0.9752 0.9774 0.9790 0.9800 0.9800 0.9800 0.9800 0.9800 0.9800 0.9800 0.9800 0.9800 0.9800 0.9800 0.9800 0.9800 0.9800 0.9800 0.9800 0.9797 0.9794 0.9790 0.9786 0.9782 0.9778 0.9774 0.9770;
      | 0.9780 0.9784 0.9787 0.9791 0.9794 0.9798 0.9800 0.9800 0.9800 0.9800 0.9800 0.9800 0.9800 0.9800 0.9800 0.9800 0.9800 0.9800 0.9800 0.9800 0.9800 0.9800 0.9799 0.9789 0.9776 0.9757 0.9730 0.9690 0.9628 0.9520 0.9301 0.8632 0.0000 0.8797 0.9347 0.9542 0.9641 0.9699 0.9737 0.9762 0.9781 0.9794 0.9800 0.9800 0.9800 0.9800 0.9800 0.9800 0.9800 0.9800 0.9800 0.9800 0.9800 0.9800 0.9800 0.9800 0.9800 0.9800 0.9800 0.9800 0.9799 0.9795 0.9792 0.9788 0.9785];
      settings: InputPortMap=u0,u1
  Abs : Abs  SaturateOnIntegerOverflow=off
  Add{,1..3} (4 alike) : Sum
  Add4 : Sum  Inputs=-+
  Constant : Constant
  Constant1 : Constant  Value=0
  Constant10 : Constant  Value=-400
  Constant11 : Constant  Value=400
  Constant12 : Constant  Value=0
  Constant13 : Constant  Value=0
  Constant2 : Constant  Value=400
  Constant3 : Constant  Value=-400
  Constant4 : Constant  Value=-400
  Constant5 : Constant  Value=400
  Delay : Delay  DelayLength=1
  Delay1 : Delay  DelayLength=1
  Delay2 : Delay  DelayLength=1
  Display1 : Display
  Display2 : Display
  Display3 : Display
  Divide{,1,3..4} (4 alike) : Product  Inputs=*/
  Divide2 : Product  Inputs=/*
  First-Order Filter : spsFirstOrderFilterLib/First-Order Filter  FilterType=Lowpass  Tc=1  Ts=0  Initialize=off  Vac_Init=[0, 0, 60]  Vdc_Init=0  PlotResponse=off  FreqRange="[0,  200,  1]"
  Gain : Gain  Gain=-1
  Gain1 : Gain  Gain=2*pi/60
  Gain2 : Gain  Gain=2*pi/60
  Gain3 : Gain  Gain=1/1000
  Gain4 : Gain  Gain=1/8.2
  Gain5 : Gain  Gain=1/8.2
  Gain6 : Gain  Gain=2*pi/60
  Gain7 : Gain  Gain=-1
  Max{,1..3,5,7,9,12..13} (9 alike) : MinMax  Function=max  Inputs=2
  Max{4,6,8,10..11,14} (6 alike) : MinMax  Inputs=2
  Maximum_Mech_Brake_Torque : Constant  Value=-500
  Min : MinMax  Inputs=3
  Min1 : MinMax  Inputs=3
  Min2 : MinMax  Function=max  Inputs=3
  Min3 : MinMax  Function=max  Inputs=2
  Min4 : MinMax  Function=max  Inputs=3
  Min5 : MinMax  Inputs=2
  Motor_RPM_Delayed1 : InportShadow  Port=7
  Product{,1..6} (7 alike) : Product
  RPM_small : Constant
  Rate Transition : RateTransition
  Rate Transition1 : RateTransition
  Rate Transition2 : RateTransition
  Relational Operator : RelationalOperator  OutDataTypeStr=boolean  RndMeth=Simplest  InputSameDT=off
  Scope4 : Scope
      settings: ActiveDisplayYMinimum=-1  ActiveDisplayYMaximum=1  DataLoggingVariableName=ScopeData5
  Switch{,1..3,5} (5 alike) : Switch  Criteria=u2 > Threshold  SaturateOnIntegerOverflow=off  InputSameDT=off
  Switch4 : Switch  Criteria=u2 ~= 0  SaturateOnIntegerOverflow=off  InputSameDT=off
  V_Bus1 : InportShadow  Port=2
  efficiency1 : Constant  Value=0.95
  efficiency2 : Constant  Value=0.95
  efficiency3 : Constant
  efficiency4 : Constant  Value=0.95
  efficiency5 : Constant
  efficiency6 : Constant
  zero : Constant  Value=0
  Available Torque : Outport
  Driveline Torque : Outport  Port=2
  Motor_Torque_Act : Outport  Port=3
  tag scope: Mechanical_Power=global
  wires:
  Min2/1 -> Relational Operator/1, Add4/1, Switch3/3  "Motor Torque Negative Available"
  Product4/1 -> Divide3/1
  Rate Transition1/1 -> Min4/2, Min/2, Available Torque/1  "Available_Torque"
  Switch1/1 -> Scope4/1, Driveline Torque/1
  Battery2_ChrgCurrLim/1 -> Gain5/1
  Motor_RPM_Delayed/1 -> Gain1/1, 1-D Lookup Table2/1, Abs/1, 1-D Lookup Table1/1
  Min1/1 -> Switch3/1  "Motor Torque Positive Available"
  Max14/1 -> Divide3/2, Product5/2
  Max5/1 -> Min1/3, Display1/1
  Divide2/1 -> Max3/1
  Switch2/1 -> Delay2/1  "Driveline Torque"
  Max1/1 -> Switch2/1
  Gain5/1 -> Add2/1
  Constant13/1 -> Max6/2
  Divide3/1 -> Divide2/2
  Max4/1 -> Max5/1
  Constant/1 -> Max/2
  V_Bus/1 -> Product3/1, Product4/1
  Maximum_Mech_Brake_Torque/1 -> Max1/2
  Constant12/1 -> Max5/2
  Max3/1 -> Max6/1
  Battery2_DischCurrLim/1 -> Gain4/1
  Gain2/1 -> Divide2/1, Divide4/2
  Product5/1 -> Divide4/1
  Add3/1 -> Switch1/3
  Abs/1 -> Max/1
  Max6/1 -> Min2/3, Display2/1
  Battery1_DischCurrLim/1 -> Add1/2
  Gain4/1 -> Add1/1
  Constant10/1 -> Max3/2
  Divide4/1 -> Max4/2
  Add4/1 -> Max1/1
  Add1/1 -> Product3/2
  Relational Operator/1 -> Switch2/2
  1-D Lookup Table1/1 -> Min1/1
  Max/1 -> 4Quadrant Efficiency Map PMSM_Inverter2/2, Gain2/1
  Constant1/1 -> Switch2/3
  Driveline Torque Request/1 -> Relational Operator/2, Add4/2, Min2/1, Switch1/2, Switch5/2, Switch3/2, Min1/2
  Delay1/1 -> Rate Transition1/1
  Switch3/1 -> Delay1/1  "Available Motor Torque"
  Constant11/1 -> Max4/1
  Product3/1 -> Display3/1, Product5/1
  1-D Lookup Table2/1 -> Gain/1
  Add2/1 -> Product4/2
  Gain/1 -> Min2/2
  Battery1_ChrgCurrLim/1 -> Add2/2
  Delay2/1 -> Rate Transition2/1
  Rate Transition2/1 -> Add3/2  "Motor Torque"
  Gain1/1 -> Product/2
  Product/1 -> Gain3/1
  Gain3/1 -> [Mechanical_Power]
  Battery1_Current/1 -> Add/1
  Battery2_Current/1 -> Add/2
  Add/1 -> Switch4/2, Product1/2, Switch/2
  V_Bus1/1 -> Product1/1
  Product1/1 -> Product2/2, Divide1/1
  Product2/1 -> Divide/1
  Gain6/1 -> Product6/1, Divide/2
  Motor_RPM_Delayed1/1 -> 4Quadrant Efficiency Map PMSM_Inverter1/2, 1-D Lookup Table4/1, 1-D Lookup Table3/1, Max2/1, 4Quadrant Efficiency Map PMSM_Inverter/2
  RPM_small/1 -> Max2/2
  Max2/1 -> Gain6/1
  Divide/1 -> Switch/1
  Max10/1 -> Product6/2
  Product6/1 -> Divide1/2
  Divide1/1 -> Switch/3
  Switch/1 -> Switch4/1
  Switch4/1 -> Delay/1, Max11/1
  zero/1 -> Switch4/3
  4Quadrant Efficiency Map PMSM_Inverter/1 -> Max7/1
  efficiency1/1 -> Max7/2
  Max7/1 -> Max8/2
  efficiency3/1 -> Max8/1
  Max8/1 -> Product2/1
  4Quadrant Efficiency Map PMSM_Inverter1/1 -> Max9/1
  efficiency5/1 -> Max10/1
  Max9/1 -> Max10/2
  efficiency4/1 -> Max9/2
  1-D Lookup Table3/1 -> Max11/2
  1-D Lookup Table4/1 -> Gain7/1
  Gain7/1 -> Max12/2
  Max11/1 -> Max12/1
  Max12/1 -> First-Order Filter/1
  Delay/1 -> Rate Transition/1
  Rate Transition/1 -> 4Quadrant Efficiency Map PMSM_Inverter1/1, 4Quadrant Efficiency Map PMSM_Inverter/1
  Switch5/1 -> Motor_Torque_Act/1, Add3/1, Switch1/1, Product/1, 4Quadrant Efficiency Map PMSM_Inverter2/1
  efficiency6/1 -> Max14/1
  efficiency2/1 -> Max13/2
  Max13/1 -> Max14/2
  4Quadrant Efficiency Map PMSM_Inverter2/1 -> Max13/1
  First-Order Filter/1 -> Min4/1, Min/1
  Constant2/1 -> Min/3
  Min/1 -> Min3/1
  Constant3/1 -> Min3/2
  Min3/1 -> Switch5/1
  Constant4/1 -> Min4/3
  Min4/1 -> Min5/1
  Constant5/1 -> Min5/2
  Min5/1 -> Switch5/3

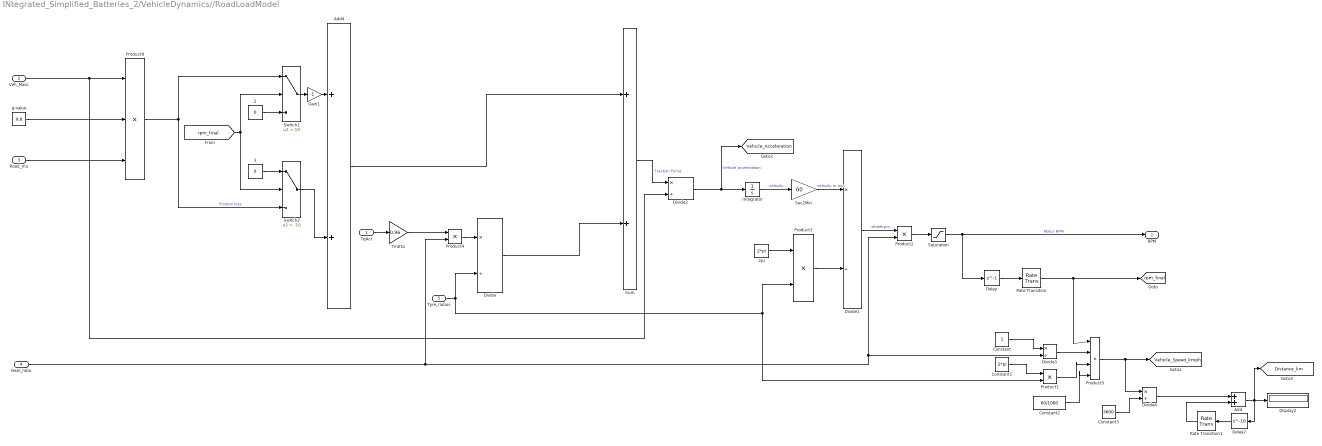
== system INtegrated_Simplified_Batteries_2/VehicleDynamics//RoadLoadModel ==
  TqAct : Inport
  Veh_Mass : Inport  Port=2
  Road_mu : Inport  Port=3
  Gear_ratio : Inport  Port=4
  Tyre_radius : Inport  Port=5
  2 : Constant  Value=0  SampleTime=-1
  2pi : Constant  Value=2*pi  SampleTime=-1
  3 : Constant  Value=0  SampleTime=-1
  Add : Sum
  Add4 : Sum
  Constant : Constant
  Constant1 : Constant  Value=2*pi
  Constant2 : Constant  Value=60/1000
  Constant3 : Constant  Value=3600
  Delay : Delay  DelayLength=1
  Delay2 : Delay  DelayLength=10
  Display2 : Display
  Divide{,1..4} (5 alike) : Product  Inputs=*/
  Gain1 : Gain  Gain=-1
  Integrator : Integrator
  Product{1..4} (4 alike) : Product
  Product5 : Product  Inputs=4
  Product9 : Product  Inputs=3
  Rate Transition : RateTransition
  Rate Transition1 : RateTransition
  Saturation : Saturate  UpperLimit=30000  LowerLimit=0
  Sec2Min : Gain  Gain=60
  Sum : Sum
  Switch1 : Switch  Criteria=u2 > Threshold  Threshold=10  SaturateOnIntegerOverflow=off  InputSameDT=off
  Switch2 : Switch  Criteria=u2 > Threshold  Threshold=-10  SaturateOnIntegerOverflow=off  InputSameDT=off
  TmEta : Gain  Gain=0.96
  g-value : Constant  Value=9.8  SampleTime=-1
  RPM : Outport
  tag scope: Distance_km=global, Vehicle_Acceleration=global, Vehicle_Speed_kmph=global, rpm_final=global
  wires:
  Road_mu/1 -> Product9/3
  Divide/1 -> Sum/2
  Product3/1 -> Divide1/2
  Tyre_radius/1 -> Product1/2, Product3/2, Divide/2
  Product4/1 -> Divide/1
  Divide2/1 -> [Vehicle_Acceleration], Integrator/1  "Vehicle acceleration"
  Sum/1 -> Divide2/1  "Traction Force"
  Integrator/1 -> Sec2Min/1  "velocity"
  2pi/1 -> Product3/1
  TqAct/1 -> TmEta/1
  Sec2Min/1 -> Divide1/1  "velocity in min"
  Divide1/1 -> Product2/1  "wheelrpm"
  Veh_Mass/1 -> Divide2/2, Product9/1
  g-value/1 -> Product9/2
  Product2/1 -> Saturation/1
  Switch1/1 -> Gain1/1
  2/1 -> Switch1/3
  Product9/1 -> Switch1/1, Switch2/3  "Friction loss"
  [rpm_final] -> Switch1/2, Switch2/2
  Switch2/1 -> Add4/2
  3/1 -> Switch2/1
  Gain1/1 -> Add4/1
  Add4/1 -> Sum/1
  Gear_ratio/1 -> Product4/2, Divide3/2, Product2/2
  TmEta/1 -> Product4/1
  Saturation/1 -> Delay/1, RPM/1  "Motor RPM"
  Delay/1 -> Rate Transition/1
  Rate Transition/1 -> Product5/1, [rpm_final]
  Constant/1 -> Divide3/1
  Constant1/1 -> Product1/1
  Divide3/1 -> Product5/2
  Product1/1 -> Product5/3
  Constant2/1 -> Product5/4
  Product5/1 -> Divide4/1, [Vehicle_Speed_kmph]
  Constant3/1 -> Divide4/2
  Divide4/1 -> Add/1
  Add/1 -> [Distance_km], Display2/1, Delay2/1
  Delay2/1 -> Rate Transition1/1
  Rate Transition1/1 -> Add/2

== system INtegrated_Simplified_Batteries_2/Battery1/Module3 ==
  Module_Current : Inport
  SubModule_1 : Subsystem
  Module_Voltage : Outport
  Module_avg_Temp : Outport  Port=2
  wires:
  SubModule_1/2(SubModule_avg_temp) -> Module_avg_Temp/1
  [Module_Current] -> SubModule_1/1(Module_Current)
  SubModule_1/1(SubModule_Voltage) -> Module_Voltage/1
  Module_Current/1 -> [Module_Current]

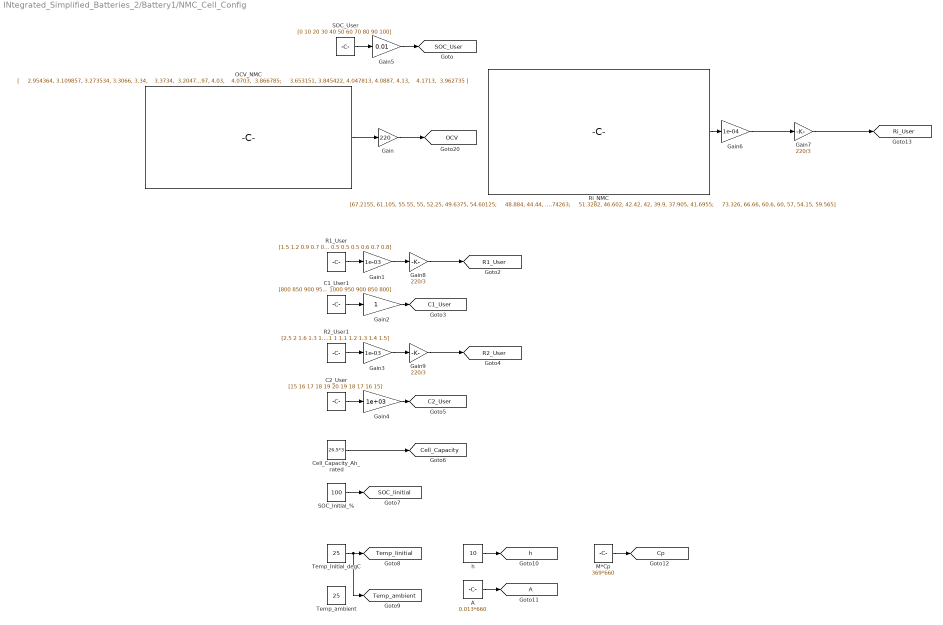
== system INtegrated_Simplified_Batteries_2/Battery1/NMC_Cell_Config ==
  A : Constant  Value=0.013*660
  C1_User1 : Constant  Value=[800 850 900 950 1000 1050 1000 950 900 850 800]
  C2_User : Constant  Value=[15 16 17 18 19 20 19 18 17 16 15]
  Cell_Capacity_Ah_rated : Constant  Value=26.5*3
  Gain : Gain  Gain=220
  Gain1 : Gain  Gain=1e-03
  Gain2 : Gain
  Gain3 : Gain  Gain=1e-03
  Gain4 : Gain  Gain=1e+03
  Gain5 : Gain  Gain=0.01
  Gain6 : Gain  Gain=1e-04
  Gain7 : Gain  Gain=220/3
  Gain8 : Gain  Gain=220/3
  Gain9 : Gain  Gain=220/3
  Goto11 : Goto  TagVisibility=global
  M*Cp : Constant  Value=369*660
  OCV_NMC : Constant  Value=|
      | [
      |     2.954364, 3.109857, 3.273534, 3.3066, 3.34,    3.3734,  3.20473;
      |     3.122427, 3.286765, 3.459753, 3.4947, 3.53,    3.5653,  3.387035;
      |     3.175499, 3.342631, 3.518559, 3.5541, 3.59,    3.6259,  3.444605;
      |     3.210881, 3.379875, 3.557763, 3.5937, 3.63,    3.6663,  3.482985;
      |     3.237417, 3.407808, 3.587166, 3.6234, 3.66,    3.6966,  3.511777;
      |     3.272799, 3.445052, 3.62637,  3.663,  3.7,     3.737,   3.55015;
      |     3.317026, 3.491066, 3.675375, 3.7125, 3.75,    3.7875,  3.598125;
      |     3.387789, 3.566094, 3.753783, 3.7917, 3.83,    3.8683,  3.674885;
      |     3.467398, 3.649892, 3.841992, 3.8808, 3.92,    3.9592,  3.76124;
      |     3.564697, 3.752313, 3.949803, 3.9897, 4.03,    4.0703,  3.866785;
      |     3.653151, 3.845422, 4.047813, 4.0887, 4.13,    4.1713,  3.962735
      | ]
  R1_User : Constant  Value=[1.5 1.2 0.9 0.7 0.6 0.5 0.5 0.5 0.6 0.7 0.8]
  R2_User1 : Constant  Value=[2.5 2 1.6 1.3 1.1 1 1.1 1.2 1.3 1.4 1.5]
  Ri_NMC : Constant  Value=|
      | [67.2155, 61.105, 55.55, 55, 52.25, 49.6375, 54.60125;
      |     48.884, 44.44, 40.4, 40, 38, 36.1, 39.71;
      |     44.60665, 40.5515, 36.865, 36.5, 34.675, 32.94125, 36.23538;
      |     41.5514, 37.774, 34.34, 34, 32.83, 30.685, 33.7535;
      |     40.3293, 36.663, 33.33, 33, 31.35, 29.7825, 32.76075;
      |     39.71825, 36.1075, 32.825, 32.5, 31.25, 29.33125, 32.26438;
      |     40.08488, 36.4408, 33.128, 32.8, 31.16, 29.602, 32.5622;
      |     40.94035, 37.2185, 33.835, 33.5, 31.825, 30.23375, 33.15738;
      |     42.7735, 38.1925, 35.03, 34.7, 32.375, 31.5875, 34.74263;
      |     51.3282, 46.602, 42.42, 42, 39.9, 37.905, 41.6955;
      |     73.326, 66.66, 60.6, 60, 57, 54.15, 59.565]
  SOC_Initial_% : Constant  Value=100
  SOC_User : Constant  Value=[0 10 20 30 40 50 60 70 80 90 100]
  Temp_Initial_degC : Constant  Value=25
  Temp_ambient : Constant  Value=25
  h : Constant  Value=10
  tag scope: C1_User=global, C2_User=global, Cell_Capacity=global, Cp=global, OCV=global, R1_User=global, R2_User=global, Ri_User=global, SOC_Iinitial=global, SOC_User=global, Temp_Iinitial=global, Temp_ambient=global, h=global
  wires:
  OCV_NMC/1 -> Gain/1
  SOC_User/1 -> Gain5/1
  R1_User/1 -> Gain1/1
  Gain1/1 -> Gain8/1
  C1_User1/1 -> Gain2/1
  Gain2/1 -> [C1_User]
  R2_User1/1 -> Gain3/1
  Gain3/1 -> Gain9/1
  Gain4/1 -> [C2_User]
  C2_User/1 -> Gain4/1
  Cell_Capacity_Ah_rated/1 -> [Cell_Capacity]
  SOC_Initial_%/1 -> [SOC_Iinitial]
  Gain5/1 -> [SOC_User]
  Temp_Initial_degC/1 -> [Temp_ambient], [Temp_Iinitial]
  h/1 -> [h]
  A/1 -> Goto11/1
  M*Cp/1 -> [Cp]
  Gain6/1 -> Gain7/1
  Ri_NMC/1 -> Gain6/1
  Gain/1 -> [OCV]
  Gain7/1 -> [Ri_User]
  Gain8/1 -> [R1_User]
  Gain9/1 -> [R2_User]

== system INtegrated_Simplified_Batteries_2/Battery1/SOCEstimator ==
  SOC_Initial : Inport
  Pack_Capacity : Inport  Port=2
  Current : Inport  Port=3
  SOCEstimator : Subsystem
  SOC : Outport
  wires:
  SOCEstimator/1(SOC) -> SOC/1
  SOC_Initial/1 -> SOCEstimator/1(SOC_Initial)
  Current/1 -> SOCEstimator/2(Current)
  Pack_Capacity/1 -> SOCEstimator/3(CellCapacity)
